simulink model "CT_CPC3_nivel"  (Simulink 8.1)
settings: Solver=ode45  StartTime=0.0  StopTime=30  FixedStep=Tm  RelTol=1e-3
InitFcn:
  | Tm = 0.01;
settings Model: Creator=Equipo-Servo  LastModifiedBy=Equipo-Servo  ExtModeTrigDuration=100000
settings DataIOCC: SignalLoggingSaveFormat=Dataset
settings OptimizationCC: ExpressionDepthLimit=128
settings DebuggingCC: FcnCallInpInsideContextMsg=EnableAllAsError
settings HardwareCC: ProdIntDivRoundTo=Zero  ProdEndianess=LittleEndian  ProdHWDeviceType=Generic->32-bit x86 compatible
settings RTWCC: SystemTargetFile=rtwin.tlc  TemplateMakefile=rtwin.tmf  Description=Real-Time Windows Target  ProcessScript=rtwin_make_rtw_hook  RTWCompilerOptimization=On
settings CodeAppCC: MaxIdLength=95
settings RTWinTargetCC: TargetLibSuffix=_rtwin.lib  TargetPreCompLibLocation=C:\Program Files\MATLAB\R2013a\toolbox\rtw\targets\rtwin\lib\win32  CodeReplacementLibrary=ANSI_C  RTWinDir=C:/PROGRA~1/MATLAB/R2013a/toolbox/rtw/targets/rtwin  TargetArch=win32

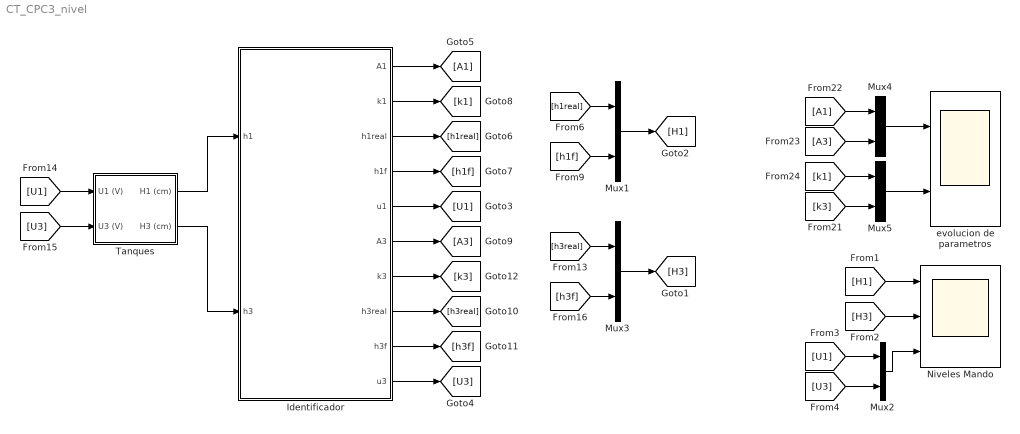
== system CT_CPC3_nivel ==
  Identificador : Subsystem
  Mux{1..5} (5 alike) : Mux  Inputs=2
  Niveles Mando : Scope  NumInputPorts=3
      settings: TimeRange=60  YMin=4~7~0  YMax=17~15.5~5
  Tanques : Subsystem
  evolucion de parametros : Scope  NumInputPorts=2
      settings: TimeRange=30  YMin=-8500~-7000  YMax=1500~1000  SaveName=parameters
  wires:
  [U1] -> Tanques/1(U1 (V))
  [U3] -> Tanques/2(U3 (V))
  Tanques/1(H1 (cm)) -> Identificador/1(h1)
  Tanques/2(H3 (cm)) -> Identificador/2(h3)
  Mux1/1 -> [H1]
  Identificador/5(u1) -> [U1]
  Identificador/10(u3) -> [U3]
  Identificador/1(A1) -> [A1]
  Identificador/3(h1real) -> [h1real]
  Identificador/4(h1f) -> [h1f]
  Mux3/1 -> [H3]
  Identificador/6(A3) -> [A3]
  Identificador/8(h3real) -> [h3real]
  Identificador/9(h3f) -> [h3f]
  [h1f] -> Mux1/2
  [h1real] -> Mux1/1
  Identificador/2(k1) -> [k1]
  Identificador/7(k3) -> [k3]
  [h3f] -> Mux3/2
  [h3real] -> Mux3/1
  [H1] -> Niveles Mando/1
  [H3] -> Niveles Mando/2
  [U1] -> Mux2/1
  [U3] -> Mux2/2
  Mux2/1 -> Niveles Mando/3
  [A1] -> Mux4/1
  [A3] -> Mux4/2
  [k1] -> Mux5/1
  [k3] -> Mux5/2
  Mux5/1 -> evolucion de parametros/2
  Mux4/1 -> evolucion de parametros/1

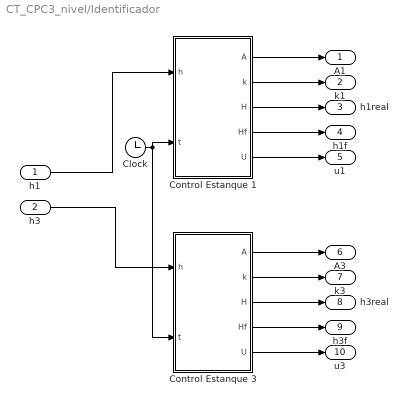
== system CT_CPC3_nivel/Identificador ==
  h1 : Inport
  h3 : Inport  Port=2
  Clock : Clock
  Control Estanque 1 : MATLAB Function  TreatAsAtomicUnit=on
  Control Estanque 3 : MATLAB Function  TreatAsAtomicUnit=on
  A1 : Outport
  k1 : Outport  Port=2
  h1real : Outport  Port=3
  h1f : Outport  Port=4
  u1 : Outport  Port=5
  A3 : Outport  Port=6
  k3 : Outport  Port=7
  h3real : Outport  Port=8
  h3f : Outport  Port=9
  u3 : Outport  Port=10
  wires:
  h3/1 -> Control Estanque 3/1(h)
  h1/1 -> Control Estanque 1/1(h)
  Control Estanque 1/1(A) -> A1/1
  Control Estanque 1/3(H) -> h1real/1
  Control Estanque 1/4(Hf) -> h1f/1
  Control Estanque 1/5(U) -> u1/1
  Control Estanque 3/1(A) -> A3/1
  Control Estanque 3/3(H) -> h3real/1
  Control Estanque 3/4(Hf) -> h3f/1
  Control Estanque 3/5(U) -> u3/1
  Clock/1 -> Control Estanque 1/2(t), Control Estanque 3/2(t)
  Control Estanque 1/2(k) -> k1/1
  Control Estanque 3/2(k) -> k3/1

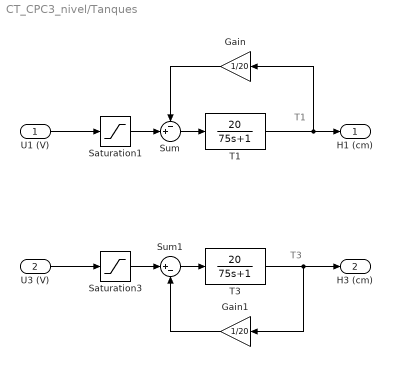
== system CT_CPC3_nivel/Tanques ==
  note: T3
  note: T1
  U1 (V) : Inport
  U3 (V) : Inport  Port=2
  Gain : Gain  Gain=1/20
  Gain1 : Gain  Gain=1/20
  Saturation1 : Saturate  UpperLimit=5  LowerLimit=0
  Saturation3 : Saturate  UpperLimit=5  LowerLimit=0
  Sum : Sum  Inputs=-+|
  Sum1 : Sum  Inputs=|+-
  T1 : TransferFcn  Numerator=[20]  Denominator=[75 1]
  T3 : TransferFcn  Numerator=[20]  Denominator=[75 1]
  H1 (cm) : Outport
  H3 (cm) : Outport  Port=2
  wires:
  T1/1 -> Gain/1, H1 (cm)/1
  U1 (V)/1 -> Saturation1/1
  U3 (V)/1 -> Saturation3/1
  T3/1 -> Gain1/1, H3 (cm)/1
  Saturation1/1 -> Sum/2
  Sum/1 -> T1/1
  Gain/1 -> Sum/1
  Saturation3/1 -> Sum1/1
  Sum1/1 -> T3/1
  Gain1/1 -> Sum1/2

== matlab function Identificador/Control Estanque 3 ==
  data: h input double; A output double; k output double; H output double; Hf output double; U output double; t input double
function [A,k,H,Hf,U] = fcn(h,t)

Tm = 0.5;
alpha = exp(-1*Tm);
persistent h1f h1f1 theta u1k1 P count a fe
if isempty(h1f)
    h1f = 0;
    h1f1= 0;
    u1k1 = 0;
    theta = ones(2,1);
    P = 1e3*eye(2);
    count = 0;
    a = 0;
    fe = 0;
end

%% entrada en volts [0, 5] V
if (t >= 10*count), fe = 5*a; a = 1 - a; count = count + 1;end

U = fe;

%% filtro de primer orden
h1f = alpha*h1f + (1 - alpha)*h;

%% Indetificador de Parametros mínimos cuadrados recursivos
u1k = U;
theta(:,1) = [1;1];
A = Tm*25/theta(1,1);
k = A*theta(2,1)/Tm;

h1f1 = h1f;
u1k1 = u1k;

%% salidas
H = h;
Hf = h1f;

== matlab function Identificador/Control Estanque 1 ==
  data: h input double; A output double; k output double; H output double; Hf output double; U output double; t input double
function [A,k,H,Hf,U] = fcn(h,t)

Tm = 0.5;
alpha = exp(-1*Tm);
persistent h1f h1f1 theta u1k1 P count a fe
if isempty(h1f)
    h1f = 0;
    h1f1= 0;
    u1k1 = 0;
    theta = ones(2,1);
    P = 1e3*eye(2);
    count = 0;
    a = 1;
    fe = 5;
end

%% entrada en volts [0, 5] V
if (t >= 10*count), fe = 5*a; a = 1 - a; count = count + 1;end

U = fe;

%% filtro de primer orden
h1f = alpha*h1f + (1 - alpha)*h;

%% Indetificador de Parametros mínimos cuadrados recursivos
u1k = U;

theta(:,1) = [1;1];

A = Tm*25/theta(1,1);
k = A*theta(2,1)/Tm;

h1f1 = h1f;
u1k1 = u1k;

%% salidas
H = h;
Hf = h1f;
